simulink model "lab4_2"  (R2018a)
settings: Solver=VariableStepAuto  StartTime=0.0  StopTime=10.0  RelTol=1e-3
settings Model: Creator=Yan Tszyafen  LastModifiedBy=Yan Tszyafen

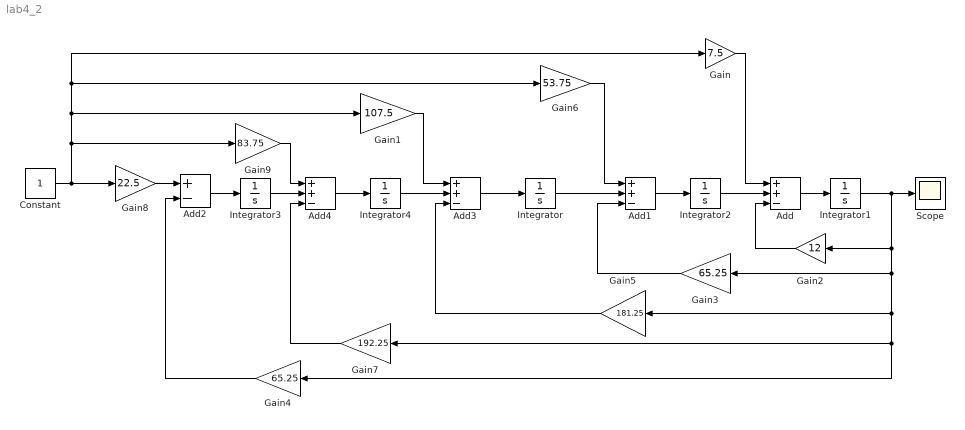
== system lab4_2 ==
  Add{,1,3..4} (4 alike) : Sum  Inputs=++-
  Add2 : Sum  Inputs=+-
  Constant : Constant
  Gain : Gain  Gain=7.5
  Gain1 : Gain  Gain=107.5
  Gain2 : Gain  Gain=12
  Gain3 : Gain  Gain=65.25
  Gain4 : Gain  Gain=65.25
  Gain5 : Gain  Gain=181.25
  Gain6 : Gain  Gain=53.75
  Gain7 : Gain  Gain=192.25
  Gain8 : Gain  Gain=22.5
  Gain9 : Gain  Gain=83.75
  Integrator{,1..4} (5 alike) : Integrator
  Scope : Scope
  wires:
  Integrator1/1 -> Gain4/1, Gain7/1, Gain5/1, Gain3/1, Gain2/1, Scope/1
  Add/1 -> Integrator1/1
  Integrator2/1 -> Add/2
  Gain/1 -> Add/1
  Gain2/1 -> Add/3
  Add1/1 -> Integrator2/1
  Integrator/1 -> Add1/2
  Gain3/1 -> Add1/3
  Gain6/1 -> Add1/1
  Add3/1 -> Integrator/1
  Integrator4/1 -> Add3/2
  Gain1/1 -> Add3/1
  Gain5/1 -> Add3/3
  Add4/1 -> Integrator4/1
  Add2/1 -> Integrator3/1
  Integrator3/1 -> Add4/2
  Gain7/1 -> Add4/3
  Gain9/1 -> Add4/1
  Gain4/1 -> Add2/2
  Gain8/1 -> Add2/1
  Constant/1 -> Gain/1, Gain6/1, Gain1/1, Gain9/1, Gain8/1
